simulink library "HY_General_Library"  (R2018b)
settings: Solver=ode45  StartTime=0.0  StopTime=10.0  RelTol=1e-3  EnableMultiTasking=on
undefined symbols (not defined in the file or in its folder): dT, Slope1, Slope2
libraries: simulink x63, $bdroot x4
(part 2 of 5)

== system HY_General_Library/Time&Counter_Blocks ==
  BounceTimer : Subsystem  mask(BounceTimer){}
      mask help:
      | HY Library for Function Development
      |
      | BounceTimer
      |
      | I/O
      | TmrEna: Timer enable flag
      | Inc:    Increase step
      | MaxTime:Maximum count time
      | Timer:  Count time
      | TrigOut:
      |         Count time >= Maximum time  -> 1
      |         Count time <  Maximum time  -> 0
  COUNTER : Subsystem  mask(COUNTER){mMAX=1byte}
      mask prompts: mMAX "最大计数字节 :"
      mask help:
      | 皓耘功能开发库
      |
      | 计数器
      |
      | 使能时开始计数，非使能时，自动清零
      | 最大计数值由参数界面选择，当前提供1/2/4字节可选
      |
      | 输入：
      | E：   计数使能输入（布尔型）
      | mMax：最大计数值
      |
      | 输出：
      | y：   计数值输出（无符号整型）
      mask init:
      | name=get_param(gcb,'MaskValueString');
      | mMAX=2^( str2num(name(1)) * 8 ) - 1;
      | limit_value = mMAX;
      mask TypeOptions mMAX: 1byte | 2byte | 4byte
      mask Display:
      | color('orange');
      | port_label('input',1,'E');
      | color('black');
      | port_label('output',1,'y');
      | text(0.5,0.1,sprintf('%s', char(num2str(limit_value))),'horizontalAlignment','center');
      | color('blue');
      | plot([0.2,0.3,0.3,0.4,0.4,0.5,0.5,0.6,0.6,0.7,0.7,0.8],[0.2,0.2,0.3,0.3,0.4,0.4,0.5,0.5,0.6,0.6,0.7,0.7]);
      | 
      | color('magenta');
      | text(1,0,'HY','horizontalAlignment','right','verticalAlignment','bottom');
  COUNTER_H : Subsystem  mask(COUNTER_H){mMAX=1byte}
      mask prompts: mMAX "最大计数字节 :"
      mask help:
      | 皓耘功能开发库
      |
      | 计数器（带复位保持）
      |
      | 复位使能时，计数清零，此优先级高于计数使能
      | 计数使能时，开始计数，计数非使能时，计数值保持
      | 最大计数值由参数界面选择，当前提供1/2/4字节可选
      |
      | 输入：
      | E：   计数使能输入（布尔型）
      | R：   计数清零输入（布尔型）
      | mMax：最大计数值
      |
      | 输出：
      | y：   计数值输出（无符号整型）
      mask init:
      | name=get_param(gcb,'MaskValueString');
      | mMAX=2^( str2num(name(1)) * 8 ) - 1;
      | limit_value=mMAX;
      mask TypeOptions mMAX: 1byte | 2byte | 4byte
      mask Display:
      | color('orange');
      | port_label('input',1,'E');
      | port_label('input',2,'R');
      | color('black');
      | port_label('output',1,'y');
      | text(0.5,0.1,sprintf('%s', char(num2str(limit_value))),'horizontalAlignment','center');
      | color('blue');
      | plot([0.2,0.3,0.3,0.4,0.4,0.5,0.5,0.6,0.6,0.7,0.7,0.8],[0.2,0.2,0.3,0.3,0.4,0.4,0.5,0.5,0.5,0.5,0.6,0.6]);
      | text(0.5,0.6,'H');
      | 
      | color('magenta');
      | text(1,0,'HY','horizontalAlignment','right','verticalAlignment','bottom');
  STOPWATCH_RE : Subsystem  Description=""  mask(STOPWATCH_RE){}
      mask help:
      | HY Library for Function Development
      |
      | I/O
      | E: start flag
      |    1 : timer count up
      |    0 : timer hold
      | R: reset timer
      |    1 : timer clear
      |    0 : None
      | dT:delta time
      |
      | t: count time
      |
      | The block outputs the time since the system init or the last reset.
      settings: AttributesFormatString=TIMER
      mask Display:
      | color('orange');
      | port_label('input',1,'E');
      | port_label('input',2,'R');
      | 
      | color('black');
      | port_label('input',3,'dT');
      | port_label('output',1,'t');
      | 
      | plot(0.5+0.35*cos(0:pi/12:2*pi),0.5+0.35*sin(0:pi/12:2*pi));
      | plot([0.5,0.5],[0.85,0.75]);
      | plot([0.5,0.5],[0.15,0.25]);
      | plot([0.15,0.25],[0.5,0.5]);
      | plot([0.75,0.85],[0.5,0.5]);
      | color('blue');
      | plot([0.5,0.5+0.25*cos(pi/4)],[0.5,0.5+0.25*sin(pi/4)]);
      | plot([0.5,0.5+0.15*cos(pi*3/2)],[0.5,0.5+0.15*sin(pi*3/2)]);
      | plot(0.5+0.01*cos(0:pi/22:2*pi),0.5+0.01*sin(0:pi/22:2*pi));
      | color('magenta');
      | text(1,0,'HY','horizontalAlignment','right','verticalAlignment','bottom');
  TIMER : Subsystem  mask(TIMER){}
      mask help:
      | HY Library for Function Development
      | Timer
      |
      | I/O
      | S: start_flag
      |    1 : timer count up
      |    0 : timer clear
      | T: target_time
      |    Target time
      | dT:delta time
      |
      | y: alarm
      |    1 : timer_value >= target_time
      |    0 : timer_value < target_time
      | t: timer_value
      |    Timer value(up count)
      settings: AttributesFormatString=TIMER
      mask Display:
      | color('orange');
      | port_label('input',2,'S');
      | port_label('output',1,'y');
      | 
      | color('black');
      | port_label('input',1,'T');
      | port_label('input',3,'dT');
      | port_label('output',2,'t');
      | 
      | plot(0.5+0.35*cos(0:pi/12:2*pi),0.5+0.35*sin(0:pi/12:2*pi));
      | plot([0.5,0.5],[0.85,0.75]);
      | plot([0.5,0.5],[0.15,0.25]);
      | plot([0.15,0.25],[0.5,0.5]);
      | plot([0.75,0.85],[0.5,0.5]);
      | color('blue');
      | plot([0.5,0.5+0.25*cos(pi/4)],[0.5,0.5+0.25*sin(pi/4)]);
      | plot([0.5,0.5+0.15*cos(pi*3/2)],[0.5,0.5+0.15*sin(pi*3/2)]);
      | plot(0.5+0.01*cos(0:pi/22:2*pi),0.5+0.01*sin(0:pi/22:2*pi));
      | text(0.3,0.5,'T');
      | color('magenta');
      | text(1,0,'HY','horizontalAlignment','right','verticalAlignment','bottom');
  TIMER_H : Subsystem  mask(TIMER_H){}
      mask help:
      | HY Library for Function Development
      |
      | Timer with holder
      | I/O
      | E: start flag
      |    1 : timer count up
      |    0 : timer hold
      | R: reset timer
      |    1 : timer clear
      |    0 : None
      | T: target time
      | dT:delta time
      |
      | y: alarm
      |    1 : timer_value >= target_time
      |    0 : timer_value < target_time
      | t:timer value
      |    Timer value(up count)
      settings: AttributesFormatString=TIMER
      mask Display:
      | color('orange');
      | port_label('input',2,'E');
      | port_label('input',3,'R');
      | port_label('output',1,'y');
      | 
      | color('black');
      | port_label('input',1,'T');
      | port_label('input',4,'dT');
      | port_label('output',2,'t');
      | 
      | plot(0.5+0.35*cos(0:pi/12:2*pi),0.5+0.35*sin(0:pi/12:2*pi));
      | plot([0.5,0.5],[0.85,0.75]);
      | plot([0.5,0.5],[0.15,0.25]);
      | plot([0.15,0.25],[0.5,0.5]);
      | plot([0.75,0.85],[0.5,0.5]);
      | color('blue');
      | plot([0.5,0.5+0.25*cos(pi/4)],[0.5,0.5+0.25*sin(pi/4)]);
      | plot([0.5,0.5+0.15*cos(pi*3/2)],[0.5,0.5+0.15*sin(pi*3/2)]);
      | plot(0.5+0.01*cos(0:pi/22:2*pi),0.5+0.01*sin(0:pi/22:2*pi));
      | text(0.3,0.5,'T');
      | text(0.65,0.5,'H');
      | color('magenta');
      | text(1,0,'HY','horizontalAlignment','right','verticalAlignment','bottom');
  TIME_Y : Subsystem  mask(TIMER_Y){}
      mask help:
      | HY Library for Function Development
      | Timer_without t
      |
      | I/O
      | S: start_flag
      |    1 : timer count up
      |    0 : timer clear
      | T: target_time
      |    Target time
      | dT:delta time
      |
      | y: alarm
      |    1 : timer_value >= target_time
      |    0 : timer_value < target_time
      settings: AttributesFormatString=TIMER
      mask Display:
      | color('orange');
      | port_label('input',2,'S');
      | port_label('output',1,'y');
      | 
      | color('black');
      | port_label('input',1,'T');
      | port_label('input',3,'dT');
      | 
      | plot(0.5+0.35*cos(0:pi/12:2*pi),0.5+0.35*sin(0:pi/12:2*pi));
      | plot([0.5,0.5],[0.85,0.75]);
      | plot([0.5,0.5],[0.15,0.25]);
      | plot([0.15,0.25],[0.5,0.5]);
      | plot([0.75,0.85],[0.5,0.5]);
      | color('blue');
      | plot([0.5,0.5+0.25*cos(pi/4)],[0.5,0.5+0.25*sin(pi/4)]);
      | plot([0.5,0.5+0.15*cos(pi*3/2)],[0.5,0.5+0.15*sin(pi*3/2)]);
      | plot(0.5+0.01*cos(0:pi/22:2*pi),0.5+0.01*sin(0:pi/22:2*pi));
      | text(0.3,0.5,'T');
      | color('magenta');
      | text(1,0,'HY','horizontalAlignment','right','verticalAlignment','bottom');
  TurnOffDelay : Subsystem  mask(TurnOffDelay){}
      mask help:
      | 皓耘功能开发库
      |
      | 基于时间的关闭延时器
      |
      | 输入：
      | u：  开关状态输入（布尔型）
      | T：  延时时间输入（浮点型）
      | dT： 模块运行周期输入（浮点型）
      |
      | 输出：
      | y：  开关状态输出（布尔型）
      mask Display:
      | color('orange');
      | plot([0.25,0.65,0.65],[0.7,0.7,0.3]);
      | port_label('input',1,'u');
      | port_label('output',1,'y');
      | color('black');
      | port_label('input',2,'T');
      | port_label('input',3,'dT');
      | 
      | color('blue');
      | plot([0.15,0.25],[0.7,0.7]);
      | plot([0.25,0.25],[0.3,0.4]);
      | plot([0.25,0.25],[0.45,0.55]);
      | plot([0.25,0.25],[0.6,0.7]);
      | plot([0.25,0.3],[0.3,0.3]);
      | plot([0.35,0.4],[0.3,0.3]);
      | plot([0.45,0.5],[0.3,0.3]);
      | plot([0.55,0.6],[0.3,0.3]);
      | plot([0.65,0.85],[0.3,0.3]);
      | plot([0.22 0.25],[0.53 0.46]);
      | plot([0.25 0.28],[0.46 0.53]);
      | text(0.45,0.50,'T')
      | 
      | color('magenta');
      | text(1,0,'HY','horizontalAlignment','right','verticalAlignment','bottom');
  TurnOffDelayCnt : Subsystem  mask(TurnOffDelayCnt){}
      mask help:
      | 皓耘功能开发库
      |
      | 基于计数的关闭延时器
      |
      | 输入：
      | u：  开关状态输入（布尔型）
      | Cnt：延时最大计数输入（无符号整型）
      |
      | 输出：
      | y：  开关状态输出（布尔型）
      mask Display:
      | color('orange');
      | plot([0.25,0.65,0.65],[0.7,0.7,0.3]);
      | port_label('input',1,'u');
      | port_label('output',1,'y');
      | color('black');
      | port_label('input',2,'Cnt');
      | 
      | color('blue');
      | plot([0.15,0.25],[0.7,0.7]);
      | plot([0.25,0.25],[0.3,0.4]);
      | plot([0.25,0.25],[0.45,0.55]);
      | plot([0.25,0.25],[0.6,0.7]);
      | plot([0.25,0.3],[0.3,0.3]);
      | plot([0.35,0.4],[0.3,0.3]);
      | plot([0.45,0.5],[0.3,0.3]);
      | plot([0.55,0.6],[0.3,0.3]);
      | plot([0.65,0.85],[0.3,0.3]);
      | plot([0.22 0.25],[0.53 0.46]);
      | plot([0.25 0.28],[0.46 0.53]);
      | text(0.5,0.5,'Cnt','horizontalAlignment','center')
      | 
      | color('magenta');
      | text(1,0,'HY','horizontalAlignment','right','verticalAlignment','bottom');
  TurnOffDelay_R : Subsystem  mask(TurnOffDelay_R){}
      mask help:
      | 皓耘功能开发库
      |
      | 基于时间的关闭延时器（带复位）
      |
      | 输入：
      | u：  开关状态输入（布尔型）
      | R：  复位指令输入（布尔型）
      | T：  延时时间输入（浮点型）
      | dT： 模块运行周期输入（浮点型）
      |
      | 输出：
      | y：  开关状态输出（布尔型）
      |
      | 如果R等于True，y输出False
      mask Display:
      | color('orange');
      | plot([0.25,0.65,0.65],[0.7,0.7,0.3]);
      | port_label('input',1,'u');
      | port_label('input',2,'R');
      | port_label('output',1,'y');
      | color('black');
      | port_label('input',3,'T');
      | port_label('input',4,'dT');
      | 
      | color('blue');
      | plot([0.15,0.25],[0.7,0.7]);
      | plot([0.25,0.25],[0.3,0.4]);
      | plot([0.25,0.25],[0.45,0.55]);
      | plot([0.25,0.25],[0.6,0.7]);
      | plot([0.25,0.3],[0.3,0.3]);
      | plot([0.35,0.4],[0.3,0.3]);
      | plot([0.45,0.5],[0.3,0.3]);
      | plot([0.55,0.6],[0.3,0.3]);
      | plot([0.65,0.85],[0.3,0.3]);
      | plot([0.22 0.25],[0.53 0.46]);
      | plot([0.25 0.28],[0.46 0.53]);
      | text(0.45,0.50,'T')
      | 
      | color('magenta');
      | text(1,0,'HY','horizontalAlignment','right','verticalAlignment','bottom');
  TurnOnDelay : Subsystem  mask(TurnOnDelay){}
      mask help:
      | 皓耘功能开发库
      |
      | 基于时间的打开延时器
      |
      | 输入：
      | u：  开关状态输入（布尔型）
      | T：  延时时间输入（浮点型）
      | dT： 模块运行周期输入（浮点型）
      |
      | 输出：
      | y：  开关状态输出（布尔型）
      mask Display:
      | color('orange');
      | plot([0.25,0.65,0.65],[0.3,0.3,0.7]);
      | port_label('input',1,'u');
      | port_label('output',1,'y');
      | color('black');
      | port_label('input',2,'T');
      | port_label('input',3,'dT');
      | 
      | color('blue');
      | plot([0.15,0.25],[0.3,0.3]);
      | plot([0.25,0.25],[0.3,0.4]);
      | plot([0.25,0.25],[0.45,0.55]);
      | plot([0.25,0.25],[0.6,0.7]);
      | plot([0.25,0.3],[0.7,0.7]);
      | plot([0.35,0.4],[0.7,0.7]);
      | plot([0.45,0.5],[0.7,0.7]);
      | plot([0.55,0.6],[0.7,0.7]);
      | plot([0.65,0.85],[0.7,0.7]);
      | plot([0.22 0.25],[0.46 0.53]);
      | plot([0.25 0.28],[0.53 0.46]);
      | text(0.45,0.5,'T')
      | 
      | color('magenta');
      | text(1,0,'HY','horizontalAlignment','right','verticalAlignment','bottom');
  TurnOnDelayCnt : Subsystem  mask(TurnOnDelayCnt){}
      mask help:
      | 皓耘功能开发库
      |
      | 基于计数的打开延时器
      |
      | 输入：
      | u：  开关状态输入（布尔型）
      | Cnt：延时最大计数输入（无符号整型）
      |
      | 输出：
      | y：  开关状态输出（布尔型）
      mask Display:
      | color('orange');
      | plot([0.25,0.65,0.65],[0.3,0.3,0.7]);
      | port_label('input',1,'u');
      | port_label('output',1,'y');
      | color('black');
      | port_label('input',2,'Cnt');
      | 
      | color('blue');
      | plot([0.15,0.25],[0.3,0.3]);
      | plot([0.25,0.25],[0.3,0.4]);
      | plot([0.25,0.25],[0.45,0.55]);
      | plot([0.25,0.25],[0.6,0.7]);
      | plot([0.25,0.3],[0.7,0.7]);
      | plot([0.35,0.4],[0.7,0.7]);
      | plot([0.45,0.5],[0.7,0.7]);
      | plot([0.55,0.6],[0.7,0.7]);
      | plot([0.65,0.85],[0.7,0.7]);
      | plot([0.22 0.25],[0.46 0.53]);
      | plot([0.25 0.28],[0.53 0.46]);
      | text(0.5,0.5,'Cnt','horizontalAlignment','Center')
      | 
      | color('magenta');
      | text(1,0,'HY','horizontalAlignment','right','verticalAlignment','bottom');
  TurnOnDelay_IV : Subsystem  mask(TurnOnDelay){}
      mask help:
      | HY Library for Function Development
      |
      | Trun on delay
      |
      | A rising edge of the input signal u is delayed by the time T.
      |
      | I/O
      | u:  Signal input(Boolean)
      | T:  Delay time
      | dT: Detal time
      mask Display:
      | color('orange');
      | plot([0.25,0.65,0.65],[0.3,0.3,0.7]);
      | port_label('input',1,'u');
      | port_label('output',1,'y');
      | port_label('input',4,'IV');
      | color('black');
      | port_label('input',2,'T');
      | port_label('input',3,'dT');
      | 
      | color('blue');
      | plot([0.15,0.25],[0.3,0.3]);
      | plot([0.25,0.25],[0.3,0.4]);
      | plot([0.25,0.25],[0.45,0.55]);
      | plot([0.25,0.25],[0.6,0.7]);
      | plot([0.25,0.3],[0.7,0.7]);
      | plot([0.35,0.4],[0.7,0.7]);
      | plot([0.45,0.5],[0.7,0.7]);
      | plot([0.55,0.6],[0.7,0.7]);
      | plot([0.65,0.85],[0.7,0.7]);
      | plot([0.22 0.25],[0.46 0.53]);
      | plot([0.25 0.28],[0.53 0.46]);
      | text(0.45,0.5,'T')
      | 
      | color('magenta');
      | text(1,0,'HY','horizontalAlignment','right','verticalAlignment','bottom');

== system HY_General_Library/Trigger_Blocks ==
  EVENT : Subsystem  mask(EVENT){SampleTime=0.01, EventTime=0.1}
      mask prompts: SampleTime "Sample_time"; EventTime "Event_time"
      mask help:
      | HY Library for Function Development
      |
      | Down edge event : Every Event_time
      |
      | * Can not use EVENT library in triggered/enabled subsystem
      mask init:
      | name=get_param(gcb,'MaskValueString');
      | name=sprintf(strrep(name,'|','\n'));
      | name=strread(name,'%s','delimiter',',');
      mask Display:
      | port_label('output',1,'event');
      | disp(sprintf('Sample_time = %s \nEvent_time = %s', char(name(1)) , char(name(2))))
      | color('magenta');
      | text(1,0,'HY','horizontalAlignment','right','verticalAlignment','bottom');
  PWM : Subsystem  mask(PWM){}
      mask help:
      | HY Library for Function Development
      |
      | PWM EVENT OUTPUT
      |
      | Inputs:
      | E    - start PWM enable flag
      | ONT  - PWM on time
      | OFFT - PWM off time
      | dT   - sample time
      mask Display:
      | color('orange');
      | port_label('input',3,'E');
      | 
      | color('black');
      | port_label('input',1,'ONT');
      | port_label('input',2,'OFFT');
      | port_label('input',4,'dT');
      | port_label('output',1,'PWM');
      | 
      | color('blue');
      | plot([0.2,0.3,0.3,0.5,0.5,0.7,0.7,0.8],[0.3,0.3,0.7,0.7,0.3,0.3,0.7,0.7]);
      | color('magenta');
      | text(1,0,'HY','horizontalAlignment','right','verticalAlignment','bottom');

== system HY_General_Library/Algebric_Blocks/DIVIDE ==
  P : Inport
  D : Inport  Port=2
  Constant1 : Constant  Value=abs(MinRange)  OutDataTypeStr=Inherit: Inherit via back propagation
  Constant2 : Constant  Value=-abs(MinRange)  OutDataTypeStr=Inherit: Inherit via back propagation
  Constant4 : Constant  Value=0  OutDataTypeStr=Inherit: Inherit via back propagation
  Divide : Product  Inputs=*/
  Relational Operator1 : RelationalOperator  OutDataTypeStr=boolean  RndMeth=Nearest  InputSameDT=on
  Subsystem : Subsystem
  Subsystem1 : Subsystem
  Switch : Switch  Criteria=u2 ~= 0
  y : Outport
  wires:
  Constant4/1 -> Relational Operator1/2
  Divide/1 -> y/1
  Switch/1 -> Divide/2
  P/1 -> Divide/1
  D/1 -> Subsystem1/1(In1), Subsystem/1(In1), Relational Operator1/1
  Relational Operator1/1 -> Switch/2
  Constant1/1 -> Subsystem1/2(In2)
  Constant2/1 -> Subsystem/2(In2)
  Subsystem/1(MinOut) -> Switch/3
  Subsystem1/1(MaxOut) -> Switch/1

== system HY_General_Library/Algebric_Blocks/TrqPwr_Cnv ==
  u : Inport
  Spd : Inport  Port=2
  Constant : Constant  Value=9550  OutDataTypeStr=single
      settings: AttributesFormatString=%<OutDataTypeStr>
  Constant1 : Constant  Value=9550  OutDataTypeStr=single
      settings: AttributesFormatString=%<OutDataTypeStr>
  Product1 : Product  Inputs=**  SaturateOnIntegerOverflow=on  InputSameDT=on  OutDataTypeStr=Inherit: Same as first input
  Product2 : Product  Inputs=*/  SaturateOnIntegerOverflow=on  InputSameDT=on  OutDataTypeStr=Inherit: Same as first input
  Product3 : Product  Inputs=*/  SaturateOnIntegerOverflow=on  InputSameDT=on  OutDataTypeStr=Inherit: Same as first input
  Product4 : Product  Inputs=**  SaturateOnIntegerOverflow=on  InputSameDT=on  OutDataTypeStr=Inherit: Same as first input
  Switch : Switch  Criteria=u2 ~= 0  InputSameDT=on
      settings: AttributesFormatString=%<Criteria>
  Trq2Pwr : Constant  Value=Trq2Pwr
  y : Outport
  wires:
  Product1/1 -> Product3/1
  Constant1/1 -> Product4/2
  Spd/1 -> Product1/2, Product2/2
  Product2/1 -> Switch/3
  Trq2Pwr/1 -> Switch/2
  Switch/1 -> y/1
  u/1 -> Product4/1, Product1/1
  Constant/1 -> Product3/2
  Product3/1 -> Switch/1
  Product4/1 -> Product2/1

== system HY_General_Library/Algebric_Blocks/Unit_Cnv ==
  u : Inport
  Gain : Gain  Gain=g
  y : Outport
  wires:
  Gain/1 -> y/1  "y"
  u/1 -> Gain/1  "u"

== system HY_General_Library/Comparision_Blocks/Open_Interval ==
  H : Inport
  u : Inport  Port=2
  L : Inport  Port=3
  Constant : Constant  Value=sIndex
  Greater : RelationalOperator  Operator=>  OutDataTypeStr=boolean  RndMeth=Nearest  InputSameDT=on
  Greater1 : RelationalOperator  Operator=>  OutDataTypeStr=boolean  RndMeth=Nearest  InputSameDT=on
  GreaterOrEqual : RelationalOperator  OutDataTypeStr=boolean  RndMeth=Nearest  InputSameDT=on
  GreaterOrEqual1 : RelationalOperator  OutDataTypeStr=boolean  RndMeth=Nearest  InputSameDT=on
  Logical Operator{,1..3} (4 alike) : Logic  OutDataTypeStr=boolean
  Lower : RelationalOperator  Operator=<  OutDataTypeStr=boolean  RndMeth=Nearest  InputSameDT=on
  Lower1 : RelationalOperator  Operator=<  OutDataTypeStr=boolean  RndMeth=Nearest  InputSameDT=on
  LowerOrEqual : RelationalOperator  Operator=<=  OutDataTypeStr=boolean  RndMeth=Nearest  InputSameDT=on
  LowerOrEqual1 : RelationalOperator  Operator=<=  OutDataTypeStr=boolean  RndMeth=Nearest  InputSameDT=on
  Multiport Switch : MultiPortSwitch  DataPortOrder=Zero-based contiguous  Inputs=4  zeroidx=on
  y : Outport
  wires:
  Lower/1 -> Logical Operator/1
  Multiport Switch/1 -> y/1
  H/1 -> LowerOrEqual1/2, LowerOrEqual/2, Lower1/2, Lower/2
  Greater/1 -> Logical Operator/2
  u/1 -> Lower/1, Lower1/1, GreaterOrEqual/1, LowerOrEqual/1, Greater1/1, LowerOrEqual1/1, GreaterOrEqual1/1, Greater/1
  L/1 -> GreaterOrEqual1/2, Greater1/2, GreaterOrEqual/2, Greater/2
  Constant/1 -> Multiport Switch/1
  Logical Operator/1 -> Multiport Switch/2
  Logical Operator1/1 -> Multiport Switch/3
  Logical Operator2/1 -> Multiport Switch/4
  Logical Operator3/1 -> Multiport Switch/5
  Lower1/1 -> Logical Operator1/1
  GreaterOrEqual/1 -> Logical Operator1/2
  LowerOrEqual/1 -> Logical Operator2/1
  Greater1/1 -> Logical Operator2/2
  LowerOrEqual1/1 -> Logical Operator3/1
  GreaterOrEqual1/1 -> Logical Operator3/2

== system HY_General_Library/Debounce_Blocks/DebounceB ==
  u : Inport  OutDataTypeStr=boolean
  TAct : Inport  Port=2
  TDeact : Inport  Port=3
  dT : Inport  Port=4
  Constant2 : Constant  Value=InitialValue  OutDataTypeStr=boolean  SampleTime=-1
  Logical Operator : Logic  Operator=NOT  OutDataTypeStr=boolean
  RS_FF_IV_Pos : $bdroot/Memory_Blocks/RS_FF_IV_Pos
  TurnOnDelay : $bdroot/Time&Counter_Blocks/TurnOnDelay
      settings: AttributesFormatString=TurnOnDelay
  TurnOnDelay1 : $bdroot/Time&Counter_Blocks/TurnOnDelay
      settings: AttributesFormatString=TurnOnDelay
  y : Outport  OutDataTypeStr=boolean
  wires:
  Constant2/1 -> RS_FF_IV_Pos/3
  RS_FF_IV_Pos/1 -> y/1
  TurnOnDelay1/1 -> RS_FF_IV_Pos/2
  TAct/1 -> TurnOnDelay/2
  dT/1 -> TurnOnDelay1/3, TurnOnDelay/3
  TDeact/1 -> TurnOnDelay1/2
  u/1 -> TurnOnDelay/1, Logical Operator/1
  Logical Operator/1 -> TurnOnDelay1/1
  TurnOnDelay/1 -> RS_FF_IV_Pos/1

== system HY_General_Library/Debounce_Blocks/DebounceJump ==
  u : Inport
  Thd : Inport  Port=2
  ChkTi : Inport  Port=3
  dT : Inport  Port=4
  Logical Operator : Logic  Operator=OR  OutDataTypeStr=boolean
  MinMax : MinMax  Function=max  Inputs=2  SaturateOnIntegerOverflow=on  InputSameDT=on
  MinMax1 : MinMax  Inputs=2  SaturateOnIntegerOverflow=on  InputSameDT=on
  NOT : Logic  Operator=NOT  Inputs=1  AllPortsSameDT=off  OutDataTypeStr=boolean
  Relational Operator1 : RelationalOperator  OutDataTypeStr=boolean  RndMeth=Simplest  InputSameDT=on
  Subtract : Sum  Inputs=+-
  Switch : Switch  Criteria=u2 ~= 0  InputSameDT=on
      settings: AttributesFormatString=%<Criteria>
  TIMER : Subsystem  mask(TIMER){}
      mask help:
      | HY Library for Function Development
      | Timer
      |
      | I/O
      | S: start_flag
      |    1 : timer count up
      |    0 : timer clear
      | T: target_time
      |    Target time
      | dT:delta time
      |
      | y: alarm
      |    1 : timer_value >= target_time
      |    0 : timer_value < target_time
      settings: AttributesFormatString=TIMER
      mask Display:
      | color('orange');
      | port_label('input',2,'S');
      | port_label('output',1,'y');
      | 
      | color('black');
      | port_label('input',1,'T');
      | port_label('input',3,'dT');
      | 
      | plot(0.5+0.35*cos(0:pi/12:2*pi),0.5+0.35*sin(0:pi/12:2*pi));
      | plot([0.5,0.5],[0.85,0.75]);
      | plot([0.5,0.5],[0.15,0.25]);
      | plot([0.15,0.25],[0.5,0.5]);
      | plot([0.75,0.85],[0.5,0.5]);
      | color('blue');
      | plot([0.5,0.5+0.25*cos(pi/4)],[0.5,0.5+0.25*sin(pi/4)]);
      | plot([0.5,0.5+0.15*cos(pi*3/2)],[0.5,0.5+0.15*sin(pi*3/2)]);
      | plot(0.5+0.01*cos(0:pi/22:2*pi),0.5+0.01*sin(0:pi/22:2*pi));
      | text(0.3,0.5,'T');
      | color('magenta');
      | text(1,0,'HY','horizontalAlignment','right','verticalAlignment','bottom');
  Unit Delay1 : UnitDelay  SampleTime=-1
      settings: AttributesFormatString=Init: %<X0>
  y : Outport
  wires:
  dT/1 -> TIMER/3(dT)
  Subtract/1 -> Relational Operator1/1
  Thd/1 -> Relational Operator1/2
  ChkTi/1 -> TIMER/1(T)
  NOT/1 -> Logical Operator/1
  MinMax/1 -> Subtract/1
  MinMax1/1 -> Subtract/2
  Logical Operator/1 -> Switch/2
  TIMER/1(y) -> Logical Operator/2
  Switch/1 -> Unit Delay1/1, y/1
  Unit Delay1/1 -> MinMax1/2, MinMax/2, Switch/3
  Relational Operator1/1 -> NOT/1, TIMER/2(S)
  u/1 -> MinMax1/1, MinMax/1, Switch/1

== system HY_General_Library/Debounce_Blocks/Debounce_Cnt ==
  u : Inport  OutDataTypeStr=boolean
  ONCnt : Inport  Port=2
  OFFCnt : Inport  Port=3
  Constant2 : Constant  Value=InitialValue  OutDataTypeStr=boolean  SampleTime=-1
  Logical Operator : Logic  Operator=NOT  OutDataTypeStr=boolean
  RS_FF_IV_Pos : Subsystem  mask(RS_FF_IV){}
      mask help:
      | 皓耘功能开发库
      |
      | 锁存器初始值可调（正输出）
      |
      | 输入：
      | S:锁存使能
      | R:复位使能
      | IV:初始化输出
      |
      | 输出：
      | Q:锁存器输出
      |
      | 初始化值在端口输入设置
      | 复位使能优先级高于设置使能
      mask Help:
      | 初始化值在端口输入设置
      | 复位使能优先级高于设置使能
      mask Display:
      | color('orange');
      | port_label('input',1,'S');
      | port_label('input',2,'R');
      | port_label('input',3,'IV');
      | port_label('output',1,'Q');
      | 
      | color('blue');
      | disp('\fontsize{12}RS FF','texmode','on');
      | 
      | color('magenta');
      | text(1,0,'HY','horizontalAlignment','right','verticalAlignment','bottom');
  TurnOnDelayCnt : Subsystem  mask(TurnOnDelayCnt){}
      mask help:
      | 皓耘功能开发库
      |
      | 基于计数的打开延时器
      |
      | 输入：
      | u：  开关状态输入（布尔型）
      | Cnt：延时最大计数输入（无符号整型）
      |
      | 输出：
      | y：  开关状态输出（布尔型）
      mask Display:
      | color('orange');
      | plot([0.25,0.65,0.65],[0.3,0.3,0.7]);
      | port_label('input',1,'u');
      | port_label('output',1,'y');
      | color('black');
      | port_label('input',2,'Cnt');
      | 
      | color('blue');
      | plot([0.15,0.25],[0.3,0.3]);
      | plot([0.25,0.25],[0.3,0.4]);
      | plot([0.25,0.25],[0.45,0.55]);
      | plot([0.25,0.25],[0.6,0.7]);
      | plot([0.25,0.3],[0.7,0.7]);
      | plot([0.35,0.4],[0.7,0.7]);
      | plot([0.45,0.5],[0.7,0.7]);
      | plot([0.55,0.6],[0.7,0.7]);
      | plot([0.65,0.85],[0.7,0.7]);
      | plot([0.22 0.25],[0.46 0.53]);
      | plot([0.25 0.28],[0.53 0.46]);
      | text(0.5,0.5,'Cnt','horizontalAlignment','Center')
      | 
      | color('magenta');
      | text(1,0,'HY','horizontalAlignment','right','verticalAlignment','bottom');
  TurnOnDelayCnt1 : Subsystem  mask(TurnOnDelayCnt){}
      mask help:
      | 皓耘功能开发库
      |
      | 基于计数的打开延时器
      |
      | 输入：
      | u：  开关状态输入（布尔型）
      | Cnt：延时最大计数输入（无符号整型）
      |
      | 输出：
      | y：  开关状态输出（布尔型）
      mask Display:
      | color('orange');
      | plot([0.25,0.65,0.65],[0.3,0.3,0.7]);
      | port_label('input',1,'u');
      | port_label('output',1,'y');
      | color('black');
      | port_label('input',2,'Cnt');
      | 
      | color('blue');
      | plot([0.15,0.25],[0.3,0.3]);
      | plot([0.25,0.25],[0.3,0.4]);
      | plot([0.25,0.25],[0.45,0.55]);
      | plot([0.25,0.25],[0.6,0.7]);
      | plot([0.25,0.3],[0.7,0.7]);
      | plot([0.35,0.4],[0.7,0.7]);
      | plot([0.45,0.5],[0.7,0.7]);
      | plot([0.55,0.6],[0.7,0.7]);
      | plot([0.65,0.85],[0.7,0.7]);
      | plot([0.22 0.25],[0.46 0.53]);
      | plot([0.25 0.28],[0.53 0.46]);
      | text(0.5,0.5,'Cnt','horizontalAlignment','Center')
      | 
      | color('magenta');
      | text(1,0,'HY','horizontalAlignment','right','verticalAlignment','bottom');
  y : Outport  OutDataTypeStr=boolean
  wires:
  Constant2/1 -> RS_FF_IV_Pos/3(IV)
  RS_FF_IV_Pos/1(Q) -> y/1
  TurnOnDelayCnt1/1(y) -> RS_FF_IV_Pos/2(R)
  ONCnt/1 -> TurnOnDelayCnt/2(Cnt)
  OFFCnt/1 -> TurnOnDelayCnt1/2(Cnt)
  u/1 -> TurnOnDelayCnt/1(u), Logical Operator/1
  Logical Operator/1 -> TurnOnDelayCnt1/1(u)
  TurnOnDelayCnt/1(y) -> RS_FF_IV_Pos/1(S)

== system HY_General_Library/Debounce_Blocks/Debounce_OBD_FCN ==
  bErr : Inport  OutDataTypeStr=boolean
  bRst : Inport  Port=2  OutDataTypeStr=boolean
  bEna : Inport  Port=3  OutDataTypeStr=boolean  PortDimensions=1
  FailThd : Inport  Port=4  OutDataTypeStr=int16
  RecThd : Inport  Port=5  OutDataTypeStr=int16
  IncrFail : Inport  Port=6  OutDataTypeStr=int16
  DecrRec : Inport  Port=7  OutDataTypeStr=int16
  Debounce_OBD : Subsystem  TreatAsAtomicUnit=on
  Logical Operator : Logic  Operator=OR  AllPortsSameDT=off  OutDataTypeStr=boolean
  Logical Operator1 : Logic  AllPortsSameDT=off  OutDataTypeStr=boolean
  Logical Operator2 : Logic  Operator=NOT  Inputs=1  AllPortsSameDT=off  OutDataTypeStr=boolean
  Logical Operator3 : Logic  AllPortsSameDT=off  OutDataTypeStr=boolean
  Relational Operator : RelationalOperator  Operator===  OutDataTypeStr=boolean  RndMeth=Nearest
  Unit Delay : UnitDelay  SampleTime=-1
      settings: AttributesFormatString=<initial=%<X0>>
  Unit Delay2 : UnitDelay  SampleTime=-1
      settings: AttributesFormatString=<initial=%<X0>>
  bFailed : Outport
  wires:
  Unit Delay/1 -> Relational Operator/1
  Unit Delay2/1 -> Logical Operator1/1
  Logical Operator3/1 -> Logical Operator/1
  Logical Operator2/1 -> Logical Operator3/1
  bEna/1 -> Logical Operator3/2
  Logical Operator1/1 -> Logical Operator2/1
  Relational Operator/1 -> Logical Operator1/2
  Debounce_OBD/1(bOutRanged) -> Unit Delay2/1
  Logical Operator/1 -> Debounce_OBD/Enable
  RecThd/1 -> Debounce_OBD/4(RecThd)
  FailThd/1 -> Debounce_OBD/3(FailThd)
  bRst/1 -> Logical Operator/2, Debounce_OBD/2(bRst)
  bErr/1 -> Relational Operator/2, Debounce_OBD/1(bErr)
  Debounce_OBD/2(bFailed) -> Unit Delay/1, bFailed/1
  IncrFail/1 -> Debounce_OBD/5(IncrFail)
  DecrRec/1 -> Debounce_OBD/6(DecrRec)

== system HY_General_Library/Debounce_Blocks/Debounce_OBD_FCN_St ==
  bErr : Inport  OutDataTypeStr=boolean
  bRst : Inport  Port=2  OutDataTypeStr=boolean
  bEna : Inport  Port=3  OutDataTypeStr=boolean  PortDimensions=1
  FailThd : Inport  Port=4  OutDataTypeStr=int16
  RecThd : Inport  Port=5  OutDataTypeStr=int16
  IncrFail : Inport  Port=6  OutDataTypeStr=int16
  DecrRec : Inport  Port=7  OutDataTypeStr=int16
  bWarnIndAcv : Inport  Port=8  OutDataTypeStr=boolean
  Debounce_OBD : Subsystem  TreatAsAtomicUnit=on
  Logical Operator : Logic  Operator=OR  AllPortsSameDT=off  OutDataTypeStr=boolean
  Logical Operator1 : Logic  Inputs=3  AllPortsSameDT=off  OutDataTypeStr=boolean
  Logical Operator2 : Logic  Operator=NOT  Inputs=1  AllPortsSameDT=off  OutDataTypeStr=boolean
  Logical Operator3 : Logic  AllPortsSameDT=off  OutDataTypeStr=boolean
  Logical Operator5 : Logic  Operator=NOT  Inputs=1  AllPortsSameDT=off  OutDataTypeStr=boolean
  Relational Operator : RelationalOperator  Operator===  OutDataTypeStr=boolean  RndMeth=Nearest
  Unit Delay : UnitDelay  SampleTime=-1
      settings: AttributesFormatString=Init: %<X0>
  Unit Delay1 : UnitDelay  SampleTime=-1
      settings: AttributesFormatString=Init: %<X0>
  Unit Delay2 : UnitDelay  SampleTime=-1
      settings: AttributesFormatString=Init: %<X0>
  bFailed : Outport
  bTestNotCompl : Outport  Port=2
  bErrCfm : Outport  Port=3
  stDgo : Outport  Port=4
  wires:
  DecrRec/1 -> Debounce_OBD/6(DecrRec)
  IncrFail/1 -> Debounce_OBD/5(IncrFail)
  Debounce_OBD/1(bFailed) -> Unit Delay/1, bFailed/1
  bErr/1 -> Debounce_OBD/1(bErr), Relational Operator/2
  bRst/1 -> Debounce_OBD/2(bRst), Logical Operator/2
  Debounce_OBD/3(bErrCfm) -> bErrCfm/1
  Debounce_OBD/2(bTestNotCompl) -> Logical Operator5/1, bTestNotCompl/1
  FailThd/1 -> Debounce_OBD/3(FailThd)
  RecThd/1 -> Debounce_OBD/4(RecThd)
  Logical Operator/1 -> Debounce_OBD/Enable
  Debounce_OBD/4(bOutRanged) -> Unit Delay2/1
  Relational Operator/1 -> Logical Operator1/3
  Logical Operator1/1 -> Logical Operator2/1
  bEna/1 -> Logical Operator3/2
  Logical Operator2/1 -> Logical Operator3/1
  Logical Operator3/1 -> Logical Operator/1
  Logical Operator5/1 -> Unit Delay1/1
  Unit Delay2/1 -> Logical Operator1/2
  Unit Delay1/1 -> Logical Operator1/1
  Unit Delay/1 -> Relational Operator/1
  bWarnIndAcv/1 -> Debounce_OBD/7(bWarnIndAcv)
  Debounce_OBD/5(stDgo) -> stDgo/1

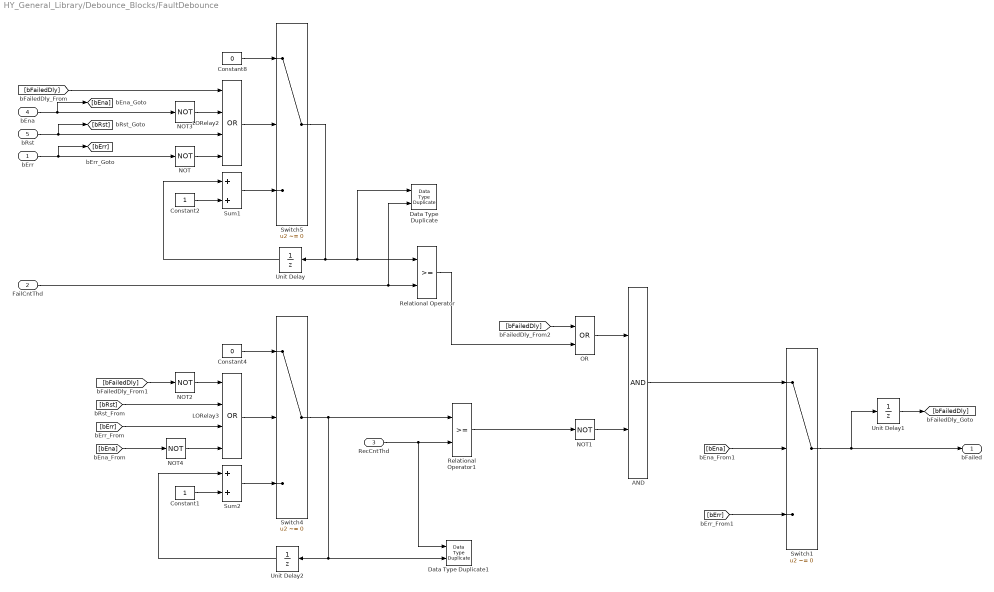
== system HY_General_Library/Debounce_Blocks/FaultDebounce ==
  bErr : Inport
  FailCntThd : Inport  Port=2
  RecCntThd : Inport  Port=3
  bEna : Inport  Port=4
  bRst : Inport  Port=5
  AND : Logic  OutDataTypeStr=boolean
  Constant1 : Constant  OutDataTypeStr=Inherit: Inherit via back propagation
  Constant2 : Constant  OutDataTypeStr=Inherit: Inherit via back propagation
  Constant4 : Constant  Value=0  OutDataTypeStr=Inherit: Inherit via back propagation
  Constant8 : Constant  Value=0  OutDataTypeStr=Inherit: Inherit via back propagation
  Data Type Duplicate : DataTypeDuplicate
  Data Type Duplicate1 : DataTypeDuplicate
  LORelay2 : Logic  Operator=OR  Inputs=4  OutDataTypeStr=boolean
  LORelay3 : Logic  Operator=OR  Inputs=4  OutDataTypeStr=boolean
  NOT{,1..4} (5 alike) : Logic  Operator=NOT  Inputs=1  AllPortsSameDT=off  OutDataTypeStr=boolean
  OR : Logic  Operator=OR  OutDataTypeStr=boolean
  Relational Operator : RelationalOperator  OutDataTypeStr=boolean  RndMeth=Simplest  InputSameDT=on
  Relational Operator1 : RelationalOperator  OutDataTypeStr=boolean  RndMeth=Simplest  InputSameDT=on
  Sum1 : Sum  OutDataTypeStr=Inherit: Inherit via back propagation  SaturateOnIntegerOverflow=on
  Sum2 : Sum  OutDataTypeStr=Inherit: Inherit via back propagation  SaturateOnIntegerOverflow=on
  Switch1 : Switch  Criteria=u2 ~= 0  SaturateOnIntegerOverflow=on  InputSameDT=on
      settings: AttributesFormatString=%<Criteria>
  Switch4 : Switch  Criteria=u2 ~= 0  SaturateOnIntegerOverflow=on  InputSameDT=on
      settings: AttributesFormatString=%<Criteria>
  Switch5 : Switch  Criteria=u2 ~= 0  SaturateOnIntegerOverflow=on  InputSameDT=on
      settings: AttributesFormatString=%<Criteria>
  Unit Delay : UnitDelay  SampleTime=-1
      settings: AttributesFormatString=Init: %<X0>
  Unit Delay1 : UnitDelay  SampleTime=-1
      settings: AttributesFormatString=Init: %<X0>
  Unit Delay2 : UnitDelay  SampleTime=-1
      settings: AttributesFormatString=Init: %<X0>
  bFailed : Outport
  wires:
  [bFailedDly] -> OR/1
  Relational Operator/1 -> OR/2
  Relational Operator1/1 -> NOT1/1
  OR/1 -> AND/1
  NOT1/1 -> AND/2
  NOT2/1 -> LORelay3/1
  Switch4/1 -> Relational Operator1/1, Data Type Duplicate1/2, Unit Delay2/1
  Unit Delay2/1 -> Sum2/1
  [bRst] -> LORelay3/2
  Constant1/1 -> Sum2/2
  Constant4/1 -> Switch4/1
  Sum2/1 -> Switch4/3
  LORelay3/1 -> Switch4/2
  [bErr] -> LORelay3/3
  [bFailedDly] -> NOT2/1
  [bFailedDly] -> LORelay2/1
  Unit Delay1/1 -> [bFailedDly]
  NOT/1 -> LORelay2/4
  LORelay2/1 -> Switch5/2
  Switch1/1 -> bFailed/1, Unit Delay1/1
  Sum1/1 -> Switch5/3
  Constant8/1 -> Switch5/1
  bErr/1 -> NOT/1, [bErr]
  Constant2/1 -> Sum1/2
  bRst/1 -> [bRst], LORelay2/3
  Unit Delay/1 -> Sum1/1
  Switch5/1 -> Unit Delay/1, Data Type Duplicate/1, Relational Operator/1
  FailCntThd/1 -> Data Type Duplicate/2, Relational Operator/2
  NOT3/1 -> LORelay2/2
  bEna/1 -> [bEna], NOT3/1
  NOT4/1 -> LORelay3/4
  [bEna] -> NOT4/1
  RecCntThd/1 -> Data Type Duplicate1/1, Relational Operator1/2
  [bEna] -> Switch1/2
  AND/1 -> Switch1/1
  [bErr] -> Switch1/3

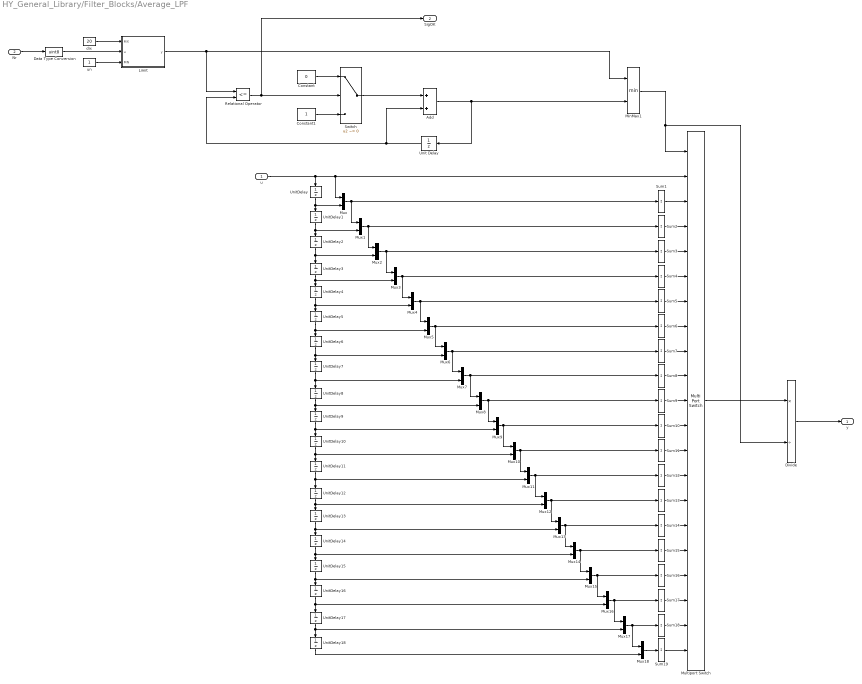
== system HY_General_Library/Filter_Blocks/Average_LPF ==
  u : Inport
  Nr : Inport  Port=2
  Add : Sum
  Constant : Constant  Value=0  OutDataTypeStr=uint8
      settings: AttributesFormatString=%<OutDataTypeStr>
  Constant1 : Constant  OutDataTypeStr=uint8
      settings: AttributesFormatString=%<OutDataTypeStr>
  Data Type Conversion : DataTypeConversion  OutDataTypeStr=uint8
  Divide : Product  Inputs=*/
  Limit : Subsystem  RTWFcnName=Limit  RTWFileName=HCU_LIB  mask(Limit){}
      settings: AttributesFormatString=Limit  RTWFcnNameOpts=User specified
      mask Display:
      | color('blue')
      | plot([0.5 0.5],[0.15 0.85],[0.2 0.8],[0.5 0.5],...
      |      [0.25,0.4,0.6,0.75],[0.25,0.25,0.75,0.75]);
      |  color('magenta');
      | text(1,0,'HY','horizontalAlignment','right','verticalAlignment','bottom');
  MinMax1 : MinMax  Inputs=2  OutDataTypeStr=uint8
  Multiport Switch : MultiPortSwitch  Inputs=20  DiagnosticForDefault=Warning  SaturateOnIntegerOverflow=on  InputSameDT=on
  Mux{,1..18} (19 alike) : Mux  Inputs=2
  Relational Operator : RelationalOperator  Operator=<=  OutDataTypeStr=boolean  RndMeth=Simplest
  Sum{1..19} (19 alike) : Sum  Inputs=+  SaturateOnIntegerOverflow=on  InputSameDT=on  OutDataTypeStr=Inherit: Same as first input
  Switch : Switch  Criteria=u2 ~= 0  InputSameDT=on
      settings: AttributesFormatString=%<Criteria>
  Unit Delay : UnitDelay  SampleTime=-1
      settings: AttributesFormatString=Init: %<X0>
  UnitDelay{,1..18} (19 alike) : UnitDelay  SampleTime=dT
      settings: AttributesFormatString=Init: %<X0>
  dix : Constant  Value=20  OutDataTypeStr=uint8
      settings: AttributesFormatString=%<OutDataTypeStr>
  un : Constant  OutDataTypeStr=uint8
      settings: AttributesFormatString=%<OutDataTypeStr>
  y : Outport
  SigOK : Outport  Port=2
  wires:
  Divide/1 -> y/1
  Sum19/1 -> Multiport Switch/21
  Mux18/1 -> Sum19/1
  UnitDelay18/1 -> Mux18/2
  Sum18/1 -> Multiport Switch/20
  Sum17/1 -> Multiport Switch/19
  Sum16/1 -> Multiport Switch/18
  Sum15/1 -> Multiport Switch/17
  Sum14/1 -> Multiport Switch/16
  Sum13/1 -> Multiport Switch/15
  Sum12/1 -> Multiport Switch/14
  Sum11/1 -> Multiport Switch/13
  Sum10/1 -> Multiport Switch/12
  Mux17/1 -> Mux18/1, Sum18/1
  UnitDelay17/1 -> UnitDelay18/1, Mux17/2
  UnitDelay14/1 -> UnitDelay15/1, Mux14/2
  Mux15/1 -> Mux16/1, Sum16/1
  Mux16/1 -> Mux17/1, Sum17/1
  UnitDelay15/1 -> UnitDelay16/1, Mux15/2
  UnitDelay16/1 -> UnitDelay17/1, Mux16/2
  Mux13/1 -> Mux14/1, Sum14/1
  Mux14/1 -> Sum15/1, Mux15/1
  UnitDelay13/1 -> UnitDelay14/1, Mux13/2
  UnitDelay10/1 -> UnitDelay11/1, Mux10/2
  Mux11/1 -> Sum12/1, Mux12/1
  Mux12/1 -> Mux13/1, Sum13/1
  UnitDelay11/1 -> UnitDelay12/1, Mux11/2
  UnitDelay12/1 -> UnitDelay13/1, Mux12/2
  Mux9/1 -> Sum10/1, Mux10/1
  Mux10/1 -> Mux11/1, Sum11/1
  UnitDelay9/1 -> UnitDelay10/1, Mux9/2
  un/1 -> Limit/3(MN)
  dix/1 -> Limit/1(MX)
  Nr/1 -> Data Type Conversion/1
  MinMax1/1 -> Multiport Switch/1, Divide/2
  Multiport Switch/1 -> Divide/1
  Mux8/1 -> Mux9/1, Sum9/1
  UnitDelay8/1 -> UnitDelay9/1, Mux8/2
  UnitDelay5/1 -> UnitDelay6/1, Mux5/2
  Mux6/1 -> Sum7/1, Mux7/1
  Mux7/1 -> Mux8/1, Sum8/1
  UnitDelay6/1 -> UnitDelay7/1, Mux6/2
  UnitDelay7/1 -> UnitDelay8/1, Mux7/2
  Mux4/1 -> Mux5/1, Sum5/1
  Mux5/1 -> Sum6/1, Mux6/1
  UnitDelay4/1 -> UnitDelay5/1, Mux4/2
  UnitDelay1/1 -> Mux1/2, UnitDelay2/1
  Mux2/1 -> Mux3/1, Sum3/1
  Mux3/1 -> Mux4/1, Sum4/1
  UnitDelay2/1 -> UnitDelay3/1, Mux2/2
  UnitDelay3/1 -> UnitDelay4/1, Mux3/2
  Sum9/1 -> Multiport Switch/11
  Sum8/1 -> Multiport Switch/10
  Sum7/1 -> Multiport Switch/9
  Sum6/1 -> Multiport Switch/8
  Sum5/1 -> Multiport Switch/7
  Sum4/1 -> Multiport Switch/6
  Sum3/1 -> Multiport Switch/5
  Sum2/1 -> Multiport Switch/4
  Sum1/1 -> Multiport Switch/3
  Mux/1 -> Sum1/1, Mux1/1
  Mux1/1 -> Mux2/1, Sum2/1
  u/1 -> UnitDelay/1, Multiport Switch/2, Mux/1
  UnitDelay/1 -> Mux/2, UnitDelay1/1
  Add/1 -> Unit Delay/1, MinMax1/2
  Switch/1 -> Add/1
  Constant1/1 -> Switch/3
  Unit Delay/1 -> Add/2, Relational Operator/2
  Limit/1(y) -> MinMax1/1, Relational Operator/1
  Relational Operator/1 -> SigOK/1, Switch/2
  Constant/1 -> Switch/1
  Data Type Conversion/1 -> Limit/2(u)

== system HY_General_Library/Filter_Blocks/DT1 ==
  u : Inport
  RV : Inport  Port=2
  R : Inport  Port=3  OutDataTypeStr=boolean
  T1 : Inport  Port=4
  dT : Inport  Port=5
  Constant : Constant  OutDataTypeStr=single  SampleTime=-1
  Divide : Product  Inputs=*/  SaturateOnIntegerOverflow=on  RndMeth=Zero  InputSameDT=on  OutDataTypeStr=Inherit: Same as first input
  Divide1 : Product  Inputs=*/  SaturateOnIntegerOverflow=on  RndMeth=Zero  InputSameDT=on  OutDataTypeStr=Inherit: Same as first input
  Divide2 : Product  Inputs=*/  SaturateOnIntegerOverflow=on  RndMeth=Zero  InputSameDT=on  OutDataTypeStr=Inherit: Same as first input
  IniCdn1 : Subsystem  mask(IniCdn){}
      mask help:
      | This block < IniCdn > is used to freeze the initial value of input signal in following way:
      | - Initial condition, output = Ini
      | - Other conditions, output = input signal
      settings: AttributesFormatString=IniCdn
      mask Display: color('blue');disp('IC')
  Sum : Sum  Inputs=++|
  Sum3 : Sum  Inputs=++-
  Switch : Switch  Criteria=u2 ~= 0  SaturateOnIntegerOverflow=on  InputSameDT=on
      settings: AttributesFormatString=threshold=%<threshold>\nCriteria : %<Criteria>
  UnitDly_ExtIni2 : Subsystem  mask(UnitDly_ExtIni){}
      mask help:
      | This block < IniCdn > is used to freeze the initial value of input signal after unit delay in following way:
      | - Initial condition, output = Ini
      | - Other conditions, output = unit delay of input signal
      mask Display:
      | color('blue')
      | dpoly(1,[1 0],'z')
  UnitDly_ExtIni3 : Subsystem  mask(UnitDly_ExtIni){}
      mask help:
      | This block < IniCdn > is used to freeze the initial value of input signal after unit delay in following way:
      | - Initial condition, output = Ini
      | - Other conditions, output = unit delay of input signal
      mask Display:
      | color('blue')
      | dpoly(1,[1 0],'z')
  product_1 : Product  SaturateOnIntegerOverflow=on  InputSameDT=on  OutDataTypeStr=Inherit: Same as first input
  product_2 : Product  SaturateOnIntegerOverflow=on  InputSameDT=on  OutDataTypeStr=Inherit: Same as first input
  product_3 : Product  SaturateOnIntegerOverflow=on  InputSameDT=on  OutDataTypeStr=Inherit: Same as first input
  y : Outport
  wires:
  IniCdn1/1(Out) -> y/1
  [RV] -> UnitDly_ExtIni2/2(RV)
  Sum3/1 -> Switch/3
  Divide2/1 -> product_2/2
  Divide1/1 -> product_3/2
  Constant/1 -> product_3/1, product_2/1
  Divide/1 -> product_1/2
  UnitDly_ExtIni3/1(Out) -> product_1/1
  UnitDly_ExtIni2/1(y) -> Divide2/1
  R/1 -> Switch/2
  product_1/1 -> Sum3/1
  product_2/1 -> Sum3/3
  product_3/1 -> Sum3/2
  u/1 -> UnitDly_ExtIni2/1(u), Divide1/1
  Sum/1 -> Divide1/2, Divide2/2, Divide/2
  dT/1 -> Sum/2
  Switch/1 -> UnitDly_ExtIni3/1(In), IniCdn1/1(In)
  T1/1 -> Sum/1, Divide/1
  RV/1 -> [RV]
  [RV] -> Switch/1
  [RV] -> IniCdn1/2(Ini)
  [RV] -> UnitDly_ExtIni3/2(Ini)

== system HY_General_Library/Filter_Blocks/LPF1_K ==
  u : Inport
  K : Inport  Port=2
  Constant : Constant  OutDataTypeStr=single
      settings: AttributesFormatString=%<OutDataTypeStr>
  Constant1 : Constant  Value=0  OutDataTypeStr=single
      settings: AttributesFormatString=%<OutDataTypeStr>
  Constant2 : Constant  OutDataTypeStr=single
      settings: AttributesFormatString=%<OutDataTypeStr>
  LIMIT : Subsystem  Description=""  mask(LIMIT){}
      mask help:
      | HY Library for Function Development
      |
      | Limits the input value u between the maximum (Max) and the minimum (Min) values.
      |
      | The input value u is checked first against the minimum value and then against the maximum value.
      |
      | In addition to that a flag is set in case the current value is higher than Max. and another flag is set in case the current value is smaller than the Min. value.
      |
      | Inputs:
      | Max  - maximum allowed value
      | Min  - minimal allowed value
      | u    - input value to be evaluated
      |
      | Output:
      | y    - limited output value
      mask Display:
      | color('black');
      | plot([0.22,0.8],[0.5,0.5]);
      | plot([0.5,0.5],[0.2,0.8]);
      | plot([0.75,0.8,0.75],[0.53,0.5,0.46]);
      | plot([0.54,0.5,0.47],[0.76,0.8,0.76]);
      | color('blue');
      | plot([0.23,0.32,0.71,0.78],[0.3,0.3,0.7,0.7]);
      | 
      | color('magenta');
      | text(1,0,'HY','horizontalAlignment','right','verticalAlignment','bottom');
  Product : Product  SaturateOnIntegerOverflow=on  RndMeth=Zero
  Product1 : Product  SaturateOnIntegerOverflow=on  RndMeth=Zero
  Subtract : Sum  SaturateOnIntegerOverflow=on
  Subtract1 : Sum  Inputs=-+  SaturateOnIntegerOverflow=on  InputSameDT=on
  Unit Delay : UnitDelay  SampleTime=-1
      settings: AttributesFormatString=Init: %<X0>
  y : Outport
  wires:
  u/1 -> Product/1
  Unit Delay/1 -> Product1/2
  Subtract/1 -> y/1, Unit Delay/1
  Product/1 -> Subtract/1
  Product1/1 -> Subtract/2
  K/1 -> LIMIT/2(u)
  Constant/1 -> LIMIT/1(Max)
  Constant1/1 -> LIMIT/3(Min)
  LIMIT/1(y) -> Subtract1/1, Product/2
  Subtract1/1 -> Product1/1
  Constant2/1 -> Subtract1/2

== system HY_General_Library/Filter_Blocks/LPF1_K_R ==
  u : Inport
  RV : Inport  Port=2
  R : Inport  Port=3
  K : Inport  Port=4
  Constant : Constant  Value=single(1)  OutDataTypeStr=single
  Constant1 : Constant  Value=single(0)  OutDataTypeStr=single
  Constant2 : Constant  Value=single(1)  OutDataTypeStr=single
  Constant3 : Constant  Value=boolean(0)  OutDataTypeStr=boolean
  LIMIT : $bdroot/Limit_Blocks/LIMIT  Description=""
  Logical Operator : Logic  Operator=OR  OutDataTypeStr=boolean
  Product : Product  SaturateOnIntegerOverflow=on  RndMeth=Zero
  Product1 : Product  SaturateOnIntegerOverflow=on  RndMeth=Zero
  Subtract : Sum  SaturateOnIntegerOverflow=on
  Subtract1 : Sum  Inputs=-+  SaturateOnIntegerOverflow=on  InputSameDT=on
  Switch : Switch  Criteria=u2 ~= 0  SaturateOnIntegerOverflow=on
      settings: AttributesFormatString=|
      | %<Criteria>
      | Threshold=%<Threshold>
  Unit Delay : UnitDelay  SampleTime=-1
      settings: AttributesFormatString=<initial=%<x0>>
  Unit Delay1 : UnitDelay  InitialCondition=1  SampleTime=-1
      settings: AttributesFormatString=<initial=%<x0>>
  y : Outport
  wires:
  R/1 -> Logical Operator/1
  RV/1 -> Switch/1
  u/1 -> Product/1
  Unit Delay/1 -> Product1/2
  Switch/1 -> Unit Delay/1, y/1
  Product/1 -> Subtract/1
  Subtract/1 -> Switch/3
  Product1/1 -> Subtract/2
  K/1 -> LIMIT/2
  Constant/1 -> LIMIT/1
  Constant1/1 -> LIMIT/3
  LIMIT/1 -> Subtract1/1, Product/2
  Subtract1/1 -> Product1/1
  Constant2/1 -> Subtract1/2
  Constant3/1 -> Unit Delay1/1
  Unit Delay1/1 -> Logical Operator/2
  Logical Operator/1 -> Switch/2

== system HY_General_Library/Filter_Blocks/LPF1_T ==
  u : Inport
  T : Inport  Port=2
  dT : Inport  Port=3
  MinMax : MinMax  Function=max  Inputs=2  SaturateOnIntegerOverflow=on  InputSameDT=on
  Product : Product  Inputs=**  SaturateOnIntegerOverflow=on  RndMeth=Zero
  Product1 : Product  Inputs=*/  SaturateOnIntegerOverflow=on  RndMeth=Zero
  Sum : Sum  SaturateOnIntegerOverflow=on
  Sum1 : Sum  Inputs=+-  SaturateOnIntegerOverflow=on
  Unit Delay : UnitDelay  SampleTime=-1
      settings: AttributesFormatString=Init: %<X0>
  y : Outport
  wires:
  MinMax/1 -> Product1/2
  T/1 -> MinMax/2
  Sum/1 -> y/1, Unit Delay/1
  Unit Delay/1 -> Sum/2, Sum1/2
  dT/1 -> MinMax/1, Product/2
  Sum1/1 -> Product/1
  Product1/1 -> Sum/1
  u/1 -> Sum1/1
  Product/1 -> Product1/1

== system HY_General_Library/Filter_Blocks/LPF1_T_R ==
  u : Inport
  RV : Inport  Port=2
  R : Inport  Port=3
  T : Inport  Port=4
  dT : Inport  Port=5
  Constant : Constant  Value=0  OutDataTypeStr=boolean
      settings: AttributesFormatString=%<OutDataTypeStr>
  K : Product  Inputs=*/  SaturateOnIntegerOverflow=on
  Logical Operator : Logic  Operator=OR  OutDataTypeStr=boolean
  MinMax : MinMax  Function=max  Inputs=2  SaturateOnIntegerOverflow=on  InputSameDT=on
  Product : Product  SaturateOnIntegerOverflow=on  RndMeth=Zero
  Subtract : Sum  SaturateOnIntegerOverflow=on
  Switch : Switch  Criteria=u2 ~= 0  SaturateOnIntegerOverflow=on  InputSameDT=on
      settings: AttributesFormatString=%<Criteria>
  Unit Delay : UnitDelay  SampleTime=-1
      settings: AttributesFormatString=Init: %<X0>
  Unit Delay1 : UnitDelay  InitialCondition=1  SampleTime=-1
      settings: AttributesFormatString=Init: %<X0>
  dif : Sum  Inputs=+-  SaturateOnIntegerOverflow=on
  y : Outport
  wires:
  Subtract/1 -> Switch/3
  dT/1 -> MinMax/1, Product/2
  T/1 -> MinMax/2
  MinMax/1 -> K/2
  K/1 -> Subtract/1
  Switch/1 -> Unit Delay/1, y/1
  Unit Delay/1 -> dif/2, Subtract/2
  dif/1 -> Product/1
  u/1 -> dif/1
  RV/1 -> Switch/1
  R/1 -> Logical Operator/1
  Product/1 -> K/1
  Logical Operator/1 -> Switch/2
  Unit Delay1/1 -> Logical Operator/2
  Constant/1 -> Unit Delay1/1

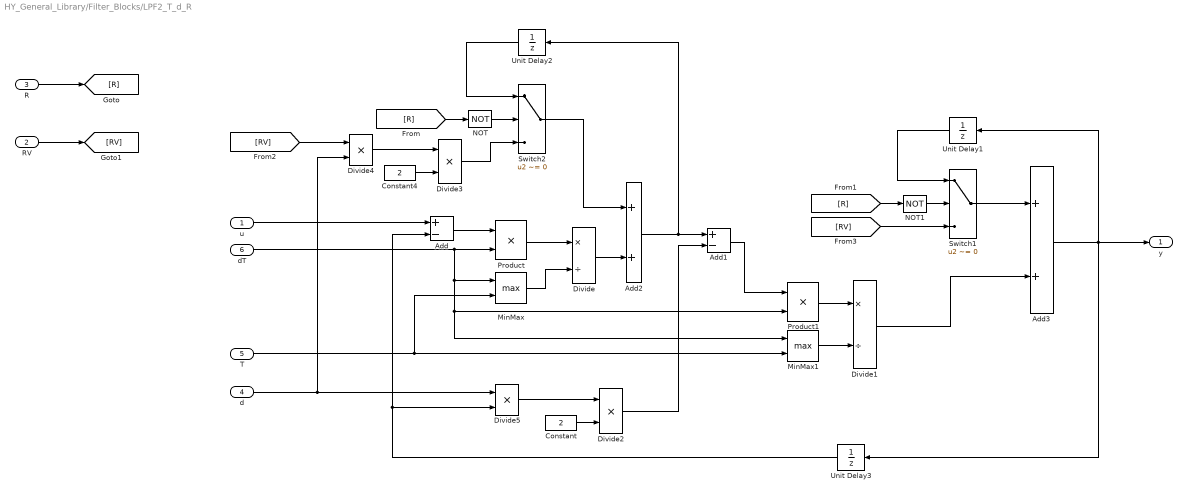
== system HY_General_Library/Filter_Blocks/LPF2_T_d_R ==
  u : Inport
  RV : Inport  Port=2
  R : Inport  Port=3
  d : Inport  Port=4
  T : Inport  Port=5
  dT : Inport  Port=6
  Add : Sum  Inputs=+-
  Add1 : Sum  Inputs=+-
  Add2 : Sum
  Add3 : Sum
  Constant : Constant  Value=2  OutDataTypeStr=single
  Constant4 : Constant  Value=2  OutDataTypeStr=single
  Divide : Product  Inputs=*/
  Divide1 : Product  Inputs=*/
  Divide{2..5} (4 alike) : Product  Inputs=**
  MinMax : MinMax  Function=max  Inputs=2  SaturateOnIntegerOverflow=on  InputSameDT=on
  MinMax1 : MinMax  Function=max  Inputs=2  SaturateOnIntegerOverflow=on  InputSameDT=on
  NOT : Logic  Operator=NOT  Inputs=1  AllPortsSameDT=off  OutDataTypeStr=boolean
  NOT1 : Logic  Operator=NOT  Inputs=1  AllPortsSameDT=off  OutDataTypeStr=boolean
  Product : Product  Inputs=**  SaturateOnIntegerOverflow=on  RndMeth=Zero
  Product1 : Product  Inputs=**  SaturateOnIntegerOverflow=on  RndMeth=Zero
  Switch1 : Switch  Criteria=u2 ~= 0
      settings: AttributesFormatString=%<Criteria>
  Switch2 : Switch  Criteria=u2 ~= 0
      settings: AttributesFormatString=%<Criteria>
  Unit Delay1 : UnitDelay  SampleTime=-1
      settings: AttributesFormatString=Init=%<X0>
  Unit Delay2 : UnitDelay  SampleTime=-1
      settings: AttributesFormatString=Init=%<X0>
  Unit Delay3 : UnitDelay  SampleTime=-1
      settings: AttributesFormatString=Init=%<X0>
  y : Outport
  wires:
  u/1 -> Add/1
  T/1 -> MinMax1/2, MinMax/2
  Divide/1 -> Add2/2
  d/1 -> Divide5/1, Divide4/2
  Constant/1 -> Divide2/2
  Divide2/1 -> Add1/2
  Add/1 -> Product/1
  dT/1 -> Product/2, MinMax1/1, Product1/2, MinMax/1
  Switch2/1 -> Add2/1
  Add2/1 -> Add1/1, Unit Delay2/1
  Add1/1 -> Product1/1
  Divide1/1 -> Add3/2
  Add3/1 -> Unit Delay3/1, Unit Delay1/1, y/1
  Unit Delay2/1 -> Switch2/1
  Switch1/1 -> Add3/1
  Unit Delay1/1 -> Switch1/1
  [R] -> NOT1/1
  [RV] -> Divide4/1
  Divide3/1 -> Switch2/3
  Constant4/1 -> Divide3/2
  [R] -> NOT/1
  R/1 -> [R]
  Unit Delay3/1 -> Add/2, Divide5/2
  Product/1 -> Divide/1
  MinMax/1 -> Divide/2
  MinMax1/1 -> Divide1/2
  Product1/1 -> Divide1/1
  Divide4/1 -> Divide3/1
  Divide5/1 -> Divide2/1
  RV/1 -> [RV]
  [RV] -> Switch1/3
  NOT/1 -> Switch2/2
  NOT1/1 -> Switch1/2

== system HY_General_Library/Hysteresis_Blocks/HysteresisA ==
  ON : Inport
  u : Inport  Port=2
  OFF : Inport  Port=3
  RESET : Constant  Value=0  OutDataTypeStr=boolean
      settings: AttributesFormatString=%<OutDataTypeStr>
  Relational Operator : RelationalOperator  Operator=<  OutDataTypeStr=boolean  RndMeth=Nearest
  Relational Operator1 : RelationalOperator  OutDataTypeStr=boolean  RndMeth=Nearest
  SET : Constant  OutDataTypeStr=boolean
      settings: AttributesFormatString=%<OutDataTypeStr>
  Switch : Switch  Criteria=u2 ~= 0  SaturateOnIntegerOverflow=on  InputSameDT=on
      settings: AttributesFormatString=%<Criteria>
  Switch1 : Switch  Criteria=u2 ~= 0  SaturateOnIntegerOverflow=on  InputSameDT=on
      settings: AttributesFormatString=%<Criteria>
  Unit Delay : UnitDelay  InitialCondition=InitialValue  SampleTime=-1
      settings: AttributesFormatString=Init: %<X0>
  y : Outport
  wires:
  OFF/1 -> Relational Operator/2
  u/1 -> Relational Operator1/1, Relational Operator/1
  ON/1 -> Relational Operator1/2
  Switch/1 -> Unit Delay/1, y/1
  Unit Delay/1 -> Switch1/3
  Switch1/1 -> Switch/3
  Relational Operator1/1 -> Switch1/2
  Relational Operator/1 -> Switch/2
  SET/1 -> Switch1/1
  RESET/1 -> Switch/1
